simulink model "New_specific_volume"  (Simulink 7.9)
settings: Solver=FixedStepDiscrete  StartTime=0.0  StopTime=0  FixedStep=1  RelTol=1e-3
undefined symbols (not defined in the file): Carnot_specific_volume_Callbacks
settings Model: DEBUGGLOBALLEVEL=1  DEBUGWRITETOFILE=0  DEBUGFILENAME=bla.txt  DEBUGMAXCONSECUTIVEWARNINGS=inf  DEBUGMAXTOTALWARNINGS=inf  Creator=awohlfei  LastModifiedBy=awohlfei

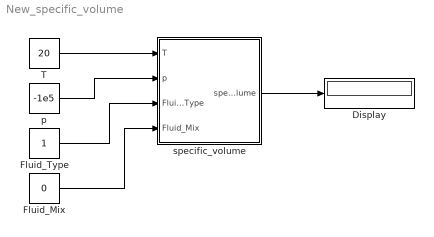
== system New_specific_volume ==
  Display : Display
  Fluid_Mix : Constant  Value=0
  Fluid_Type : Constant
  T : Constant  Value=20
  p : Constant  Value=-1e5
  specific_volume : Subsystem  LoadFcn=Carnot_specific_volume_Callbacks('LoadFcn');  InitFcn=load('THB.mat');  VariantObject=CarlibClassic  mask(specific volume){INPUTARGUMENTS=state variables (classic), DEBUGLEVEL=DEBUG, MAXTOTALWARNINGS=inf, MAXCONSECUTIVEWARNINGS=inf, WRITETOFILE=0, FILENAME='errors.txt'}
      mask prompts: INPUTARGUMENTS "Input arguments"; DEBUGLEVEL "Debug level"; MAXTOTALWARNINGS "maximum number of total warning"; MAXCONSECUTIVEWARNINGS "maximum number of consecutive warnings"; WRITETOFILE "write messages to file"; FILENAME "filename for error messages"
      mask help:
      | Calculates the specific volume of fluids [m³/kg].
      | Calls the function "specific_volume" in the CARNOT library "Carlib".
      mask init:
      | %Inports
      | Carnot_specific_volume_Callbacks('CreateInports');
      | 
      | %global debug level
      | [DEBUGLEVEL, MAXTOTALWARNINGS, MAXCONSECUTIVEWARNINGS, WRITETOFILE, FILENAME] = Carnot_specific_volume_Callbacks('CheckDebugLevels', DEBUGLEVEL, MAXTOTALWARNINGS, MAXCONSECUTIVEWARNINGS, WRITETOFILE, FILENAME);
      mask StyleString: popup(state variables (classic)|THB|THV),popup(DEBUG|INFO|WARNING|ERROR|FATAL|NONE),edit,edit,edit,edit
      mask CallbackString: Carnot_specific_volume_Callbacks('MaskVisibilities');|||||
      mask TabNameString: Parameters,Debugging,Debugging,Debugging,Debugging,Debugging
  wires:
  T/1 -> specific_volume/1(T)
  p/1 -> specific_volume/2(p)
  Fluid_Type/1 -> specific_volume/3(Fluid_Type)
  Fluid_Mix/1 -> specific_volume/4(Fluid_Mix)
  specific_volume/1(specific_volume) -> Display/1

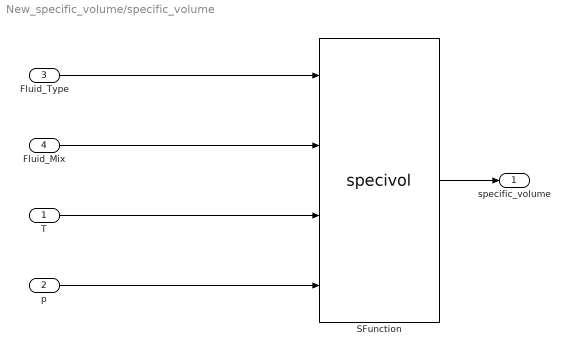
== system New_specific_volume/specific_volume ==
  T : Inport
  p : Inport  Port=2
  Fluid_Type : Inport  Port=3
  Fluid_Mix : Inport  Port=4
  SFunction : S-Function  FunctionName=specivol  Parameters=DEBUGLEVEL, MAXTOTALWARNINGS, MAXCONSECUTIVEWARNINGS, WRITETOFILE, FILENAME  EnableBusSupport=off
  specific_volume : Outport
  wires:
  SFunction/1 -> specific_volume/1
  T/1 -> SFunction/3
  p/1 -> SFunction/4
  Fluid_Type/1 -> SFunction/1
  Fluid_Mix/1 -> SFunction/2
